simulink model "doc_commmsksync"  (R2014a)
settings: Solver=FixedStepDiscrete  SolverMode=SingleTasking  StartTime=0.0  StopTime=2.0  RelTol=1e-3
model workspace (MATLAB code in the model file):
  | tsym = 1/280000;
  | sampPerSymb = 14;
  | trDepth = 16;
libraries: dspsigops x5, dspstat3 x2, commutil2 x2, simulink_extras x2, commdigbbndcpm2 x2, commsink2 x1, commblksprivate x1, commfilt2 x1, dspmathops x1, dspmtrx3 x1, commchan3 x1, commrflib2 x1
CloseFcn:
  | if exist('commmsksync_sigsOut','var'), clear commmsksync_sigsOut; end;
Description:
  | MSK Signal:  Timing, Carrier Frequency and Carrier Phase Recovery
  | 
  | This model shows the modeling of channel impairments such as timing phase offset, carrier frequency, and phase offsets for a minimum shift keying (MSK) signal.
settings Model: ExtModeAutoUpdateStatusClock=off  Creator=The MathWorks Inc.
settings DataIOCC: LimitDataPoints=off  SignalLoggingSaveFormat=ModelDataLogs  SaveOutput=off  SaveTime=off  SignalLoggingName=commmsksync_sigsOut
settings OptimizationCC: BooleanDataType=off  ExpressionDepthLimit=2147483647  InitFltsAndDblsToZero=on  EfficientMapNaN2IntZero=off
settings DebuggingCC: SaveWithParameterizedLinksMsg=none  UnderspecifiedInitializationDetection=Classic  CheckExecutionContextPreStartOutputMsg=on  CheckExecutionContextRuntimeOutputMsg=on  SignalResolutionControl=TryResolveAllWithWarning  SolverPrmCheckMsg=none  InheritedTsInSrcMsg=none  MultiTaskDSMMsg=warning  MultiTaskCondExecSysMsg=none  SigSpecEnsureSampleTimeMsg=none  FcnCallInpInsideContextMsg=UseLocalSettings  StateNameClashWarn=warning  StrictBusMsg=None
settings HardwareCC: ProdHWDeviceType=Specified
settings ModelReferenceCC: UpdateModelReferenceTargets=IfOutOfDate
settings RTWCC: IncludeERTFirstTime=on
settings GRTTargetCC: TargetFcnLib=ansi_tfl_tmw.mat  CombineOutputUpdateFcns=off  GRTInterface=on

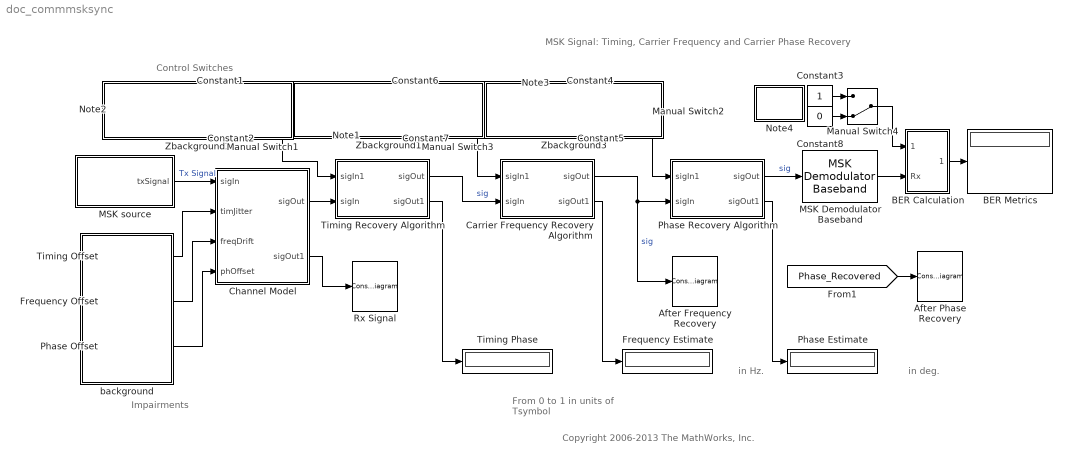
== system doc_commmsksync ==
  note: MSK Signal:
      | Timing, Carrier Frequency and Carrier Phase Recovery
  note: in Hz.
  note: From 0 to 1
      | in units of Tsymbol
  note: in deg.
  note: Control Switches
  note: Impairments
  note: Copyright 2006-2013 The MathWorks, Inc.
  After Frequency Recovery : ConstellationDiagram  Tag=ScatterPlot
  After Phase Recovery : ConstellationDiagram  Tag=ScatterPlot
  BER Calculation : Subsystem
      mask Display: disp('BER')
  BER Metrics : Display
  Carrier Frequency Recovery Algorithm : Subsystem  mask(Carrier Frequency Recovery algorithm){}
      mask Display: disp('Carrier Freq.\nRecovery')
  Channel Model : Subsystem  mask(RF Impairments){}
      mask Display: plot(-10,-10,110, 110,[05 15 10 10 05 10 18 14 13 7.5 13 41 44 47 50 53 57 59 100-[13 7.5 13 14 18 10 5 10 10 15 5]],[70 70 70 85 92 85 79 82 90 88.5 90 90 87 93 87 93 87 90 90 88.5 90 82 79 85 92 85 70 70 70]-30);
  Constant{1,3..4,6} (4 alike) : Constant  SampleTime=tsym*1000
  Constant{2,5,7..8} (4 alike) : Constant  Value=0  SampleTime=tsym*1000
  Frequency Estimate : Display
  Frequency Offset : Constant  Value=50
  MSK Demodulator Baseband : commdigbbndcpm2/MSK Demodulator Baseband  outputType=Bit  phaseOffset=0  samplesPerSymbol=1  RateOptions=Enforce single-rate processing  traceBack=trDepth  outDType=double
  MSK source : Subsystem  mask(GMSK source){}
      mask Display: disp('MSK\nSource')
  Manual Switch1 : ManualSwitch
  Manual Switch2 : ManualSwitch
  Manual Switch3 : ManualSwitch
  Manual Switch4 : ManualSwitch  CurrentSetting=0
  Note1 : Subsystem
      mask Display: disp('Carrier Frequency\nRecovery')
  Note2 : Subsystem
      mask Display: disp('Timing Phase\nRecovery')
  Note3 : Subsystem
      mask Display: disp('Phase\nRecovery')
  Note4 : Subsystem
      mask Display: disp('Reset\nBER')
  Phase Estimate : Display
  Phase Offset : Constant  Value=30
  Phase Recovery Algorithm : Subsystem  mask(Carrier Frequency Recovery algorithm){}
      mask Display: disp('Phase\nRecovery')
  Rx Signal : ConstellationDiagram  Tag=ScatterPlot
  Timing Offset : Constant  Value=0.2
  Timing Phase : Display
  Timing Recovery Algorithm : Subsystem  mask(Timing recovery algorithm.){}
      mask Display: disp('Timing\nRecovery');
  Zbackground1 : Subsystem
      mask Display: disp('')
  Zbackground2 : Subsystem
      mask Display: disp('')
  Zbackground3 : Subsystem
      mask Display: disp('')
  background : Subsystem
      mask Display: disp('')
  wires:
  Carrier Frequency Recovery Algorithm/1(sigOut) -> Phase Recovery Algorithm/2(sigIn), After Frequency Recovery/1  "sig"
  MSK source/1(txSignal) -> Channel Model/1(sigIn)  "Tx Signal"
  Channel Model/1(sigOut) -> Timing Recovery Algorithm/2(sigIn)
  Manual Switch1/1 -> Timing Recovery Algorithm/1(sigIn1)
  Timing Recovery Algorithm/1(sigOut) -> Carrier Frequency Recovery Algorithm/2(sigIn)  "sig"
  Manual Switch3/1 -> Carrier Frequency Recovery Algorithm/1(sigIn1)
  Timing Offset/1 -> Channel Model/2(timJitter)
  Frequency Offset/1 -> Channel Model/3(freqDrift)
  Timing Recovery Algorithm/2(sigOut1) -> Timing Phase/1
  Carrier Frequency Recovery Algorithm/2(sigOut1) -> Frequency Estimate/1
  Phase Recovery Algorithm/2(sigOut1) -> Phase Estimate/1
  Phase Offset/1 -> Channel Model/4(phOffset)
  Phase Recovery Algorithm/1(sigOut) -> MSK Demodulator Baseband/1  "sig"
  MSK Demodulator Baseband/1 -> BER Calculation/2(Rx)
  BER Calculation/1(Out1) -> BER Metrics/1
  Channel Model/2(sigOut1) -> Rx Signal/1
  Manual Switch4/1 -> BER Calculation/1(Rst)
  [Phase_Recovered] -> After Phase Recovery/1
  Manual Switch2/1 -> Phase Recovery Algorithm/1(sigIn1)
  Constant4/1 -> Manual Switch2/1
  Constant5/1 -> Manual Switch2/2
  Constant6/1 -> Manual Switch3/1
  Constant7/1 -> Manual Switch3/2
  Constant1/1 -> Manual Switch1/1
  Constant2/1 -> Manual Switch1/2
  Constant3/1 -> Manual Switch4/1
  Constant8/1 -> Manual Switch4/2

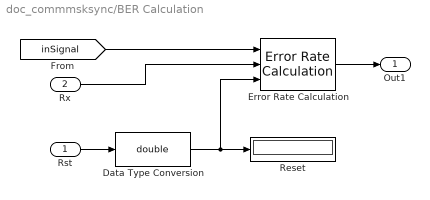
== system doc_commmsksync/BER Calculation ==
  Rst : Inport
  Rx : Inport  Port=2
  Data Type Conversion : DataTypeConversion  OutDataTypeStr=double
  Error Rate Calculation : commsink2/Error Rate Calculation  N=trDepth+2 % Traceback Depth + Delay due to Timing Recovery  st_delay=0  cp_mode=Entire frame  subframe=[]  PMode=Port  WsName=ErrorVec  RsMode2=on  stop=off  numErr=100  maxBits=1e6
  Reset : Display
  Out1 : Outport
  wires:
  Error Rate Calculation/1 -> Out1/1
  Rst/1 -> Data Type Conversion/1
  Data Type Conversion/1 -> Reset/1, Error Rate Calculation/3
  Rx/1 -> Error Rate Calculation/2
  [inSignal] -> Error Rate Calculation/1

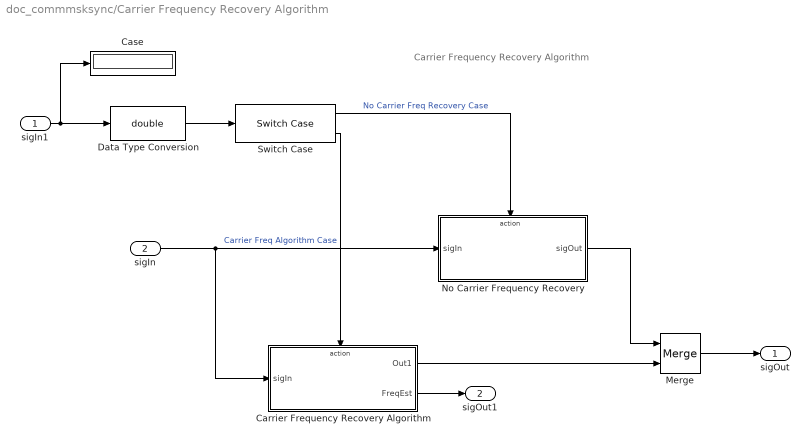
== system doc_commmsksync/Carrier Frequency Recovery Algorithm ==
  note: Carrier Frequency Recovery Algorithm
  sigIn1 : Inport
  sigIn : Inport  Port=2
  Carrier Frequency Recovery Algorithm : Subsystem  TreatAsAtomicUnit=on
  Case : Display
  Data Type Conversion : DataTypeConversion  OutDataTypeStr=double
  Merge : Merge
  No Carrier Frequency Recovery : Subsystem  TreatAsAtomicUnit=on
  Switch Case : SwitchCase  CaseConditions={0,1}  ShowDefaultCase=off
  sigOut : Outport
  sigOut1 : Outport  Port=2
  wires:
  sigIn/1 -> No Carrier Frequency Recovery/1(sigIn), Carrier Frequency Recovery Algorithm/1(sigIn)
  Merge/1 -> sigOut/1
  Switch Case/2 -> Carrier Frequency Recovery Algorithm/Action  "Carrier Freq Algorithm Case"
  Switch Case/1 -> No Carrier Frequency Recovery/Action  "No Carrier Freq Recovery Case"
  No Carrier Frequency Recovery/1(sigOut) -> Merge/1
  Carrier Frequency Recovery Algorithm/1(Out1) -> Merge/2
  Carrier Frequency Recovery Algorithm/2(FreqEst) -> sigOut1/1
  sigIn1/1 -> Data Type Conversion/1, Case/1
  Data Type Conversion/1 -> Switch Case/1

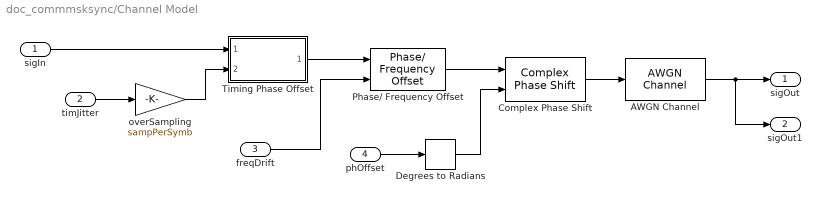
== system doc_commmsksync/Channel Model ==
  sigIn : Inport
  timJitter : Inport  Port=2
  freqDrift : Inport  Port=3
  phOffset : Inport  Port=4
  AWGN Channel : commchan3/AWGN Channel  InputProcessing=Columns as channels (frame based)  seed=67  noiseMode="Signal to noise ratio  (Eb/No)"  EbNodB=60  EsNodB=10  SNRdB=10  bitsPerSym=1  Ps=1  Tsym=tsym  variance=1
  Complex Phase Shift : commutil2/Complex Phase Shift
  Degrees to Radians : simulink_extras/Transformations/Degrees to Radians
  Phase/ Frequency Offset : commrflib2/Phase// Frequency Offset  phaseOffset=0  freqPort=on  freqOffset=0
  Timing Phase Offset : Subsystem
      mask Display: disp('Timing Phase\nOffset')
  overSampling : Gain  Gain=sampPerSymb  SaturateOnIntegerOverflow=on  OutDataTypeStr=Inherit: Same as input  ParamDataTypeStr=Inherit: Same as input
  sigOut : Outport
  sigOut1 : Outport  Port=2
  wires:
  AWGN Channel/1 -> sigOut/1, sigOut1/1
  sigIn/1 -> Timing Phase Offset/1(InSignal)
  timJitter/1 -> overSampling/1
  Timing Phase Offset/1(OutSignal) -> Phase/ Frequency Offset/1
  overSampling/1 -> Timing Phase Offset/2(phOffset)
  freqDrift/1 -> Phase/ Frequency Offset/2
  Phase/ Frequency Offset/1 -> Complex Phase Shift/1
  Complex Phase Shift/1 -> AWGN Channel/1
  Degrees to Radians/1 -> Complex Phase Shift/2
  phOffset/1 -> Degrees to Radians/1

== system doc_commmsksync/MSK source ==
  note: in bps.
  Bernoulli Binary Generator : commrandsrc2/Bernoulli Binary Generator  P=0.5  seed=61  Ts=tsym  frameBased=on  sampPerFrame=1000  orient=off  outDataType=double
  Compute Bit Rate : Subsystem  mask(Compute bit rate of signal){overSamp=sampPerSymb}
      mask prompts: overSamp "Oversampling factor:"
      mask help: Bit rate calculation based on probed sample time and a specified number of bits per sample.
      mask Display: disp('Compute\nBit Rate')
  MSK Modulator Baseband : commdigbbndcpm2/MSK Modulator Baseband  inputType=Bit  phaseOffset=0  samplesPerSymbol=sampPerSymb  RateOptions=Enforce single-rate processing  outDataType=double
  bit rate : Display
  txSignal : Outport
  tag scope: inSignal=global
  wires:
  Bernoulli Binary Generator/1 -> [inSignal], MSK Modulator Baseband/1
  MSK Modulator Baseband/1 -> Compute Bit Rate/1(sig), txSignal/1
  Compute Bit Rate/1(rate) -> bit rate/1

== system doc_commmsksync/Note1 ==

== system doc_commmsksync/Note2 ==

== system doc_commmsksync/Note3 ==

== system doc_commmsksync/Note4 ==

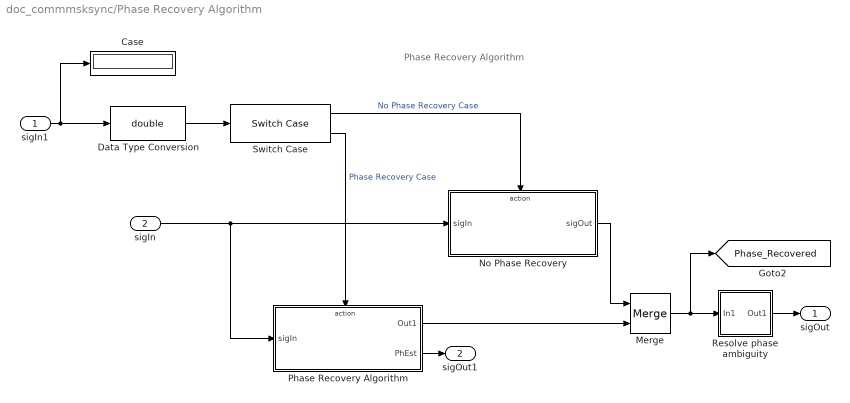
== system doc_commmsksync/Phase Recovery Algorithm ==
  note: Phase Recovery Algorithm
  sigIn1 : Inport
  sigIn : Inport  Port=2
  Case : Display
  Data Type Conversion : DataTypeConversion  OutDataTypeStr=double
  Merge : Merge
  No Phase Recovery : Subsystem  TreatAsAtomicUnit=on
  Phase Recovery Algorithm : Subsystem  TreatAsAtomicUnit=on
  Resolve phase ambiguity : Subsystem
  Switch Case : SwitchCase  CaseConditions={0,1}  ShowDefaultCase=off
  sigOut : Outport
  sigOut1 : Outport  Port=2
  tag scope: Phase_Recovered=global
  wires:
  Data Type Conversion/1 -> Switch Case/1
  sigIn1/1 -> Case/1, Data Type Conversion/1
  Phase Recovery Algorithm/2(PhEst) -> sigOut1/1
  Phase Recovery Algorithm/1(Out1) -> Merge/2
  No Phase Recovery/1(sigOut) -> Merge/1
  Switch Case/1 -> No Phase Recovery/Action  "No Phase Recovery Case"
  Switch Case/2 -> Phase Recovery Algorithm/Action  "Phase Recovery Case"
  Merge/1 -> Resolve phase ambiguity/1(In1), [Phase_Recovered]
  sigIn/1 -> Phase Recovery Algorithm/1(sigIn), No Phase Recovery/1(sigIn)
  Resolve phase ambiguity/1(Out1) -> sigOut/1

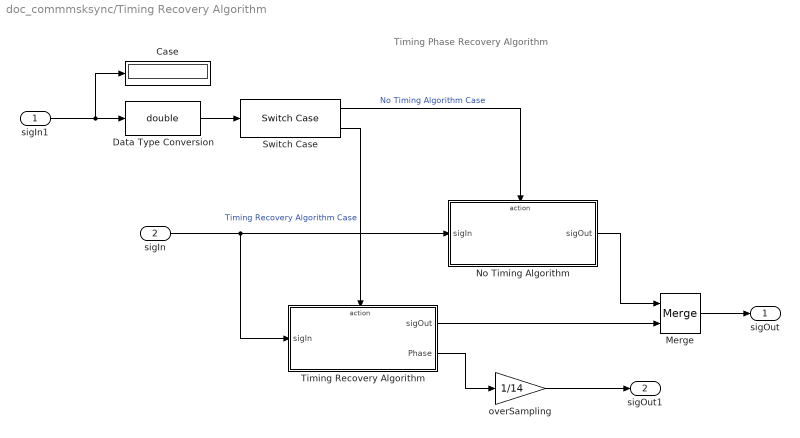
== system doc_commmsksync/Timing Recovery Algorithm ==
  note: Timing Phase Recovery Algorithm
  sigIn1 : Inport
  sigIn : Inport  Port=2
  Case : Display
  Data Type Conversion : DataTypeConversion  OutDataTypeStr=double
  Merge : Merge
  No Timing Algorithm : Subsystem  TreatAsAtomicUnit=on
  Switch Case : SwitchCase  CaseConditions={0,1}  ShowDefaultCase=off
  Timing Recovery Algorithm : Subsystem  TreatAsAtomicUnit=on
  overSampling : Gain  Gain=1/14  SaturateOnIntegerOverflow=on  OutDataTypeStr=Inherit: Same as input  ParamDataTypeStr=Inherit: Same as input
  sigOut : Outport
  sigOut1 : Outport  Port=2
  wires:
  sigIn/1 -> Timing Recovery Algorithm/1(sigIn), No Timing Algorithm/1(sigIn)
  Merge/1 -> sigOut/1
  Switch Case/2 -> Timing Recovery Algorithm/Action  "Timing Recovery Algorithm Case"
  Switch Case/1 -> No Timing Algorithm/Action  "No Timing Algorithm Case"
  No Timing Algorithm/1(sigOut) -> Merge/1
  Timing Recovery Algorithm/1(sigOut) -> Merge/2
  Timing Recovery Algorithm/2(Phase) -> overSampling/1
  sigIn1/1 -> Data Type Conversion/1, Case/1
  overSampling/1 -> sigOut1/1
  Data Type Conversion/1 -> Switch Case/1

== system doc_commmsksync/Zbackground1 ==
  note: This subsystem is empty

== system doc_commmsksync/Zbackground2 ==
  note: This subsystem is empty

== system doc_commmsksync/Zbackground3 ==
  note: This subsystem is empty

== system doc_commmsksync/background ==
  note: This subsystem is empty

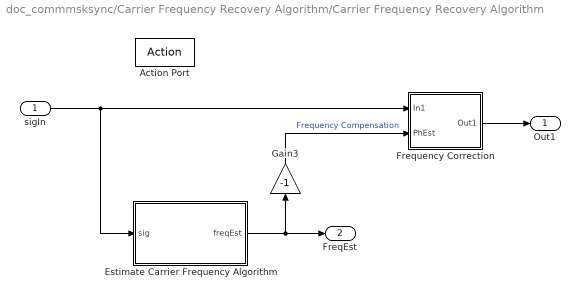
== system doc_commmsksync/Carrier Frequency Recovery Algorithm/Carrier Frequency Recovery Algorithm ==
  sigIn : Inport
  Action Port : ActionPort  InitializeStates=reset  PropagateVarSize=During execution  ActionType=case
  Estimate Carrier Frequency Algorithm : Subsystem
  Frequency Correction : Subsystem
      mask Display: disp('Frequency\nCorrection');
  Gain3 : Gain  Gain=-1  SaturateOnIntegerOverflow=on  OutDataTypeStr=Inherit: Same as input  ParamDataTypeStr=Inherit: Same as input
  Out1 : Outport
  FreqEst : Outport  Port=2  OutputWhenDisabled=reset  InitialOutput=0
  wires:
  sigIn/1 -> Estimate Carrier Frequency Algorithm/1(sig), Frequency Correction/1(In1)
  Frequency Correction/1(Out1) -> Out1/1
  Gain3/1 -> Frequency Correction/2(PhEst)  "Frequency Compensation"
  Estimate Carrier Frequency Algorithm/1(freqEst) -> FreqEst/1, Gain3/1

== system doc_commmsksync/Carrier Frequency Recovery Algorithm/No Carrier Frequency Recovery ==
  sigIn : Inport
  Action Port : ActionPort  PropagateVarSize=During execution  ActionType=case
  sigOut : Outport
  wires:
  sigIn/1 -> sigOut/1

== system doc_commmsksync/Channel Model/Timing Phase Offset ==
  InSignal : Inport
  phOffset : Inport  Port=2
  Variable Fractional Delay : dspsigops/Variable Fractional Delay  mode=OBSOLETE  modeActive=Linear  dmax=100  InputProcessing=Columns as channels (frame based)  L=4  FarrowL=4  R=10  alpha=1  ic=0  fallbackFIR=Clip to the minimum value necessary for centered kernel  fallbackFarrow=Clip to the minimum value necessary for centered kernel  noDFT=off  roundingMode=Zero  overflowMode=off
  OutSignal : Outport
  wires:
  Variable Fractional Delay/1 -> OutSignal/1
  InSignal/1 -> Variable Fractional Delay/1
  phOffset/1 -> Variable Fractional Delay/2

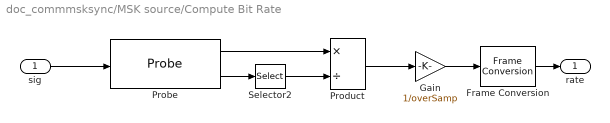
== system doc_commmsksync/MSK source/Compute Bit Rate ==
  sig : Inport
  Frame Conversion : FrameConversion
  Gain : Gain  Gain=1/overSamp  SaturateOnIntegerOverflow=on  OutDataTypeStr=Inherit: Same as input  ParamDataTypeStr=Inherit: Same as input
  Probe : Probe  ProbeComplexSignal=off
  Product : Product  Inputs=*/  SaturateOnIntegerOverflow=on  InputSameDT=on  OutDataTypeStr=Inherit: Same as first input
  Selector2 : Selector  InputPortWidth=2  Indices=[1 ]
  rate : Outport
  wires:
  Product/1 -> Gain/1
  sig/1 -> Probe/1
  Selector2/1 -> Product/2
  Probe/2 -> Selector2/1
  Probe/1 -> Product/1
  Gain/1 -> Frame Conversion/1
  Frame Conversion/1 -> rate/1

== system doc_commmsksync/Phase Recovery Algorithm/No Phase Recovery ==
  sigIn : Inport
  Action Port : ActionPort  PropagateVarSize=During execution  ActionType=case
  sigOut : Outport
  wires:
  sigIn/1 -> sigOut/1

== system doc_commmsksync/Phase Recovery Algorithm/Phase Recovery Algorithm ==
  sigIn : Inport
  Action Port : ActionPort  InitializeStates=reset  PropagateVarSize=During execution  ActionType=case
  CPM Phase Recovery : commphrec2/CPM Phase Recovery  P=2  intPeriod=1000
  Out1 : Outport
  PhEst : Outport  Port=2  OutputWhenDisabled=reset  InitialOutput=0
  wires:
  sigIn/1 -> CPM Phase Recovery/1
  CPM Phase Recovery/1 -> Out1/1
  CPM Phase Recovery/2 -> PhEst/1

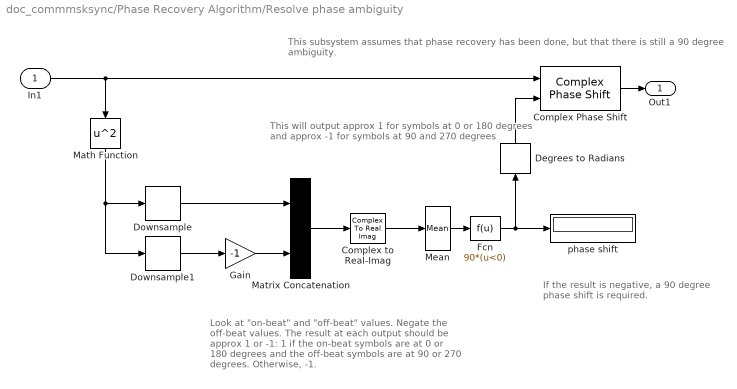
== system doc_commmsksync/Phase Recovery Algorithm/Resolve phase ambiguity ==
  note: If the result is negative,
      | a 90 degree phase shift is required.
  note: Look at "on-beat" and "off-beat" values.
      | Negate the off-beat values.
      | The result at each output should be approx 1 or -1:
      | 1 if the on-beat symbols are at 0 or 180 degrees
      | and the off-beat symbols are at 90 or 270 degrees.
      | Otherwise, -1.
  note: This will output approx 1 for symbols at 0 or 180 degrees
      | and approx -1 for symbols at 90 and 270 degrees
  note: This subsystem assumes that phase recovery has been done, but that there is still a 90 degree ambiguity.
  In1 : Inport
  Complex Phase Shift : commutil2/Complex Phase Shift
  Complex to Real-Imag : ComplexToRealImag  Output=Real
  Degrees to Radians : simulink_extras/Transformations/Degrees to Radians
  Downsample : dspsigops/Downsample  N=2  phase=0  InputProcessing=Columns as channels (frame based)  RateOptions=Enforce single-rate processing  smode=Allow multirate  fmode=Maintain input frame rate  ic=0
  Downsample1 : dspsigops/Downsample  N=2  phase=1  InputProcessing=Columns as channels (frame based)  RateOptions=Enforce single-rate processing  smode=Allow multirate  fmode=Maintain input frame rate  ic=0
  Fcn : Fcn  Expr=90*(u<0)
  Gain : Gain  Gain=-1
  Math Function : Math  Operator=square  SaturateOnIntegerOverflow=on
  Matrix Concatenation : Concatenate  Mode=Multidimensional array
  Mean : dspstat3/Mean  run=off  reset_popup=None  InputProcessing=Columns as channels (frame based)  directionMode=Each column  dimension=1  treatSBRowAsCol=on  roiEnable=off  roiType=Rectangles  roiPortion=Entire ROI  roiOutput=Individual statistics for each ROI  roiFlag=off  outputDataTypeStr=Inherit: Same as accumulator  outputLastDataTypeStr=Inherit: Same as accumulator  outputMin=[]  outputMax=[]  roundingMode=Floor  overflowMode=off
  phase shift : Display
  Out1 : Outport
  wires:
  Fcn/1 -> phase shift/1, Degrees to Radians/1
  Complex to Real-Imag/1 -> Mean/1
  Mean/1 -> Fcn/1
  Matrix Concatenation/1 -> Complex to Real-Imag/1
  Gain/1 -> Matrix Concatenation/2
  Downsample1/1 -> Gain/1
  Downsample/1 -> Matrix Concatenation/1
  Math Function/1 -> Downsample1/1, Downsample/1
  Complex Phase Shift/1 -> Out1/1
  In1/1 -> Math Function/1, Complex Phase Shift/1
  Degrees to Radians/1 -> Complex Phase Shift/2

== system doc_commmsksync/Timing Recovery Algorithm/No Timing Algorithm ==
  sigIn : Inport
  Action Port : ActionPort  PropagateVarSize=During execution  ActionType=case
  Downsample : dspsigops/Downsample  N=14  phase=0  InputProcessing=Columns as channels (frame based)  RateOptions=Enforce single-rate processing  smode=Allow multirate  fmode=Maintain input frame rate  ic=0
  sigOut : Outport
  wires:
  sigIn/1 -> Downsample/1
  Downsample/1 -> sigOut/1

== system doc_commmsksync/Timing Recovery Algorithm/Timing Recovery Algorithm ==
  note: The Sym output is the result of applying the
      | estimated phase correction to the input signal.
  note: The Ph output gives the phase estimate
      | for each symbol in the input signal.
  sigIn : Inport
  Action Port : ActionPort  InitializeStates=reset  PropagateVarSize=During execution  ActionType=case
  MSK-Type Signal Timing Recovery : commtimrec2/MSK-Type Signal Timing Recovery  modType=MSK  sampPerSymbol=sampPerSymb  propGain=0.2  resetMode=None
  Multiport Selector : dspindex/Multiport Selector  rowsOrCols=Rows  idxCellArray={1}  idxErrMode=Clip Index
  sigOut : Outport
  Phase : Outport  Port=2  OutputWhenDisabled=reset  InitialOutput=0
  wires:
  sigIn/1 -> MSK-Type Signal Timing Recovery/1
  MSK-Type Signal Timing Recovery/1 -> sigOut/1
  MSK-Type Signal Timing Recovery/2 -> Multiport Selector/1
  Multiport Selector/1 -> Phase/1

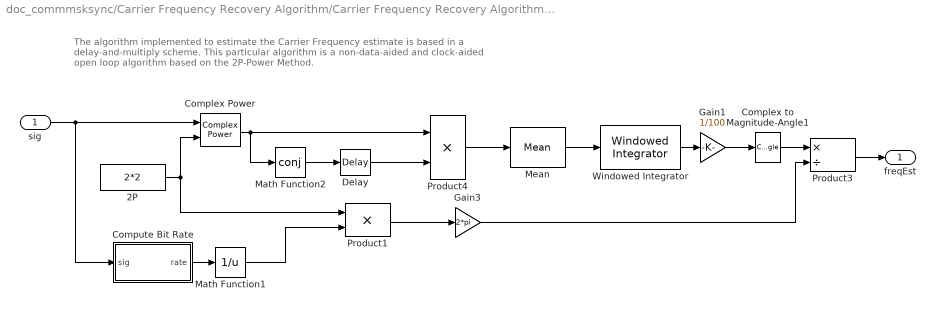
== system doc_commmsksync/Carrier Frequency Recovery Algorithm/Carrier Frequency Recovery Algorithm/Estimate Carrier Frequency Algorithm ==
  note: The algorithm implemented to estimate the Carrier Frequency estimate is based in a
      | delay-and-multiply scheme. This particular algorithm is a non-data-aided
      | and clock-aided open loop algorithm based on the 2P-Power Method.
  sig : Inport
  2P : Constant  Value=2*2
  Complex Power : commblksprivate/Complex Power
  Complex to Magnitude-Angle1 : ComplexToMagnitudeAngle  Output=Angle
  Compute Bit Rate : Subsystem  mask(Compute bit rate of signal){overSamp=1}
      mask prompts: overSamp "Oversampling factor:"
      mask help: Bit rate calculation based on probed sample time and a specified number of bits per sample.
      mask Display: disp('Compute\nBit Rate')
  Delay : dspsigops/Delay  InputProcessing=Columns as channels (frame based)  dly_unit=Samples  delay=1  ic_detail=off  dif_ic_for_ch=off  dif_ic_for_dly=off  ic=0  reset_popup=None
  Gain1 : Gain  Gain=1/100  SaturateOnIntegerOverflow=on  OutDataTypeStr=Inherit: Same as input  ParamDataTypeStr=Inherit: Same as input
  Gain3 : Gain  Gain=2*pi  SaturateOnIntegerOverflow=on  OutDataTypeStr=Inherit: Same as input  ParamDataTypeStr=Inherit: Same as input
  Math Function1 : Math  Operator=reciprocal  SaturateOnIntegerOverflow=on
  Math Function2 : Math  Operator=conj  SaturateOnIntegerOverflow=on
  Mean : dspstat3/Mean  run=off  reset_popup=None  InputProcessing=Columns as channels (frame based)  directionMode=Each column  dimension=1  treatSBRowAsCol=on  roiEnable=off  roiType=Rectangles  roiPortion=Entire ROI  roiOutput=Individual statistics for each ROI  roiFlag=off  outputDataTypeStr=Inherit: Same as accumulator  outputLastDataTypeStr=Inherit: Same as accumulator  outputMin=[]  outputMax=[]  roundingMode=Floor  overflowMode=off
  Product1 : Product  Inputs=**  SaturateOnIntegerOverflow=on  OutDataTypeStr=Inherit: Same as first input
  Product3 : Product  Inputs=*/  SaturateOnIntegerOverflow=on  OutDataTypeStr=Inherit: Same as first input
  Product4 : Product  SaturateOnIntegerOverflow=on  OutDataTypeStr=Inherit: Same as first input
  Windowed Integrator : commfilt2/Windowed Integrator  integperiod=100  roundingMode=Floor  overflowMode=off  InputProcessing=Columns as channels (frame based)
  freqEst : Outport
  wires:
  Product1/1 -> Gain3/1
  2P/1 -> Product1/1, Complex Power/2
  Complex Power/1 -> Product4/1, Math Function2/1
  Math Function2/1 -> Delay/1
  Delay/1 -> Product4/2
  Product4/1 -> Mean/1
  Complex to Magnitude-Angle1/1 -> Product3/1
  Gain3/1 -> Product3/2
  sig/1 -> Compute Bit Rate/1(sig), Complex Power/1
  Product3/1 -> freqEst/1
  Mean/1 -> Windowed Integrator/1
  Compute Bit Rate/1(rate) -> Math Function1/1
  Math Function1/1 -> Product1/2
  Gain1/1 -> Complex to Magnitude-Angle1/1
  Windowed Integrator/1 -> Gain1/1

== system doc_commmsksync/Carrier Frequency Recovery Algorithm/Carrier Frequency Recovery Algorithm/Frequency Correction ==
  In1 : Inport
  PhEst : Inport  Port=2
  Calculate Frequency Offset : Subsystem
      mask Display: disp('Calculate\nFrequency\nOffset');
  Product : Product  SaturateOnIntegerOverflow=on  InputSameDT=on  OutDataTypeStr=Inherit: Same as first input
  Out1 : Outport
  wires:
  Calculate Frequency Offset/1(Out1) -> Product/2
  In1/1 -> Calculate Frequency Offset/1(In1), Product/1
  Product/1 -> Out1/1
  PhEst/1 -> Calculate Frequency Offset/2(Freq)

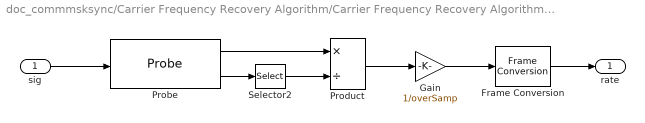
== system doc_commmsksync/Carrier Frequency Recovery Algorithm/Carrier Frequency Recovery Algorithm/Estimate Carrier Frequency Algorithm/Compute Bit Rate ==
  sig : Inport
  Frame Conversion : FrameConversion
  Gain : Gain  Gain=1/overSamp  SaturateOnIntegerOverflow=on  OutDataTypeStr=Inherit: Same as input  ParamDataTypeStr=Inherit: Same as input
  Probe : Probe  ProbeComplexSignal=off
  Product : Product  Inputs=*/  SaturateOnIntegerOverflow=on  InputSameDT=on  OutDataTypeStr=Inherit: Same as first input
  Selector2 : Selector  InputPortWidth=2  Indices=[1 ]
  rate : Outport
  wires:
  Product/1 -> Gain/1
  sig/1 -> Probe/1
  Selector2/1 -> Product/2
  Probe/2 -> Selector2/1
  Probe/1 -> Product/1
  Gain/1 -> Frame Conversion/1
  Frame Conversion/1 -> rate/1

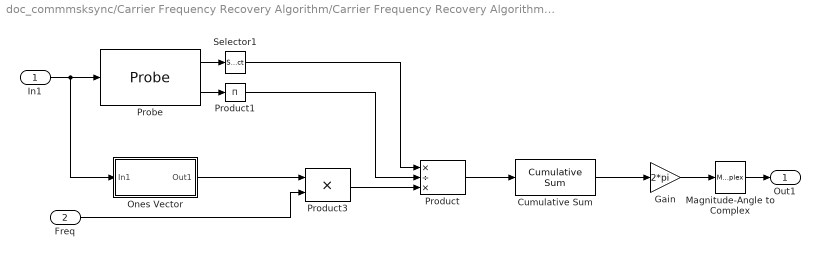
== system doc_commmsksync/Carrier Frequency Recovery Algorithm/Carrier Frequency Recovery Algorithm/Frequency Correction/Calculate Frequency Offset ==
  In1 : Inport
  Freq : Inport  Port=2
  Cumulative Sum : dspmathops/Cumulative Sum  dim=Channels (running sum)  InputProcessing=Columns as channels (frame based)  reset_popup=None  outputDataTypeStr=Inherit: Same as accumulator  outputLastDataTypeStr=Inherit: Same as accumulator  outputMin=[]  outputMax=[]  roundingMode=Floor  overflowMode=off
  Gain : Gain  Gain=2*pi  SaturateOnIntegerOverflow=on  OutDataTypeStr=Inherit: Same as input  ParamDataTypeStr=Inherit: Same as input
  Magnitude-Angle to Complex : MagnitudeAngleToComplex  Input=Angle  ConstantPart=1
  Ones Vector : Subsystem  mask(Ones Vector){}
      mask help: Create a vector of equals whose length is equal to input portwidth.
      mask Display: disp('Ones(1:length)')
  Probe : Probe  ProbeWidth=off  ProbeComplexSignal=off  ProbeSignalDimensions=on
  Product : Product  Inputs=*/*  SaturateOnIntegerOverflow=on  InputSameDT=on  OutDataTypeStr=Inherit: Same as first input
  Product1 : Product  Inputs=1  SaturateOnIntegerOverflow=on  InputSameDT=on  OutDataTypeStr=Inherit: Same as first input
  Product3 : Product  Inputs=**  SaturateOnIntegerOverflow=on  OutDataTypeStr=Inherit: Same as first input
  Selector1 : Selector  InputPortWidth=2  Indices=[1 ]
  Out1 : Outport
  wires:
  Selector1/1 -> Product/1
  Product1/1 -> Product/2
  Probe/1 -> Selector1/1
  Product/1 -> Cumulative Sum/1
  Probe/2 -> Product1/1
  In1/1 -> Probe/1, Ones Vector/1(In1)
  Magnitude-Angle to Complex/1 -> Out1/1
  Gain/1 -> Magnitude-Angle to Complex/1
  Product3/1 -> Product/3
  Freq/1 -> Product3/2
  Cumulative Sum/1 -> Gain/1
  Ones Vector/1(Out1) -> Product3/1

== system doc_commmsksync/Carrier Frequency Recovery Algorithm/Carrier Frequency Recovery Algorithm/Frequency Correction/Calculate Frequency Offset/Ones Vector ==
  In1 : Inport
  Bias : dspmtrx3/Array-Vector Add  Dimension=2  V_Source=Dialog parameter  V_VectFromMask=1  firstCoeffSignedness=Auto  firstCoeffDataTypeStr=Inherit: Same word length as input  firstCoeffLastDataTypeStr=Inherit: Same word length as input  firstCoeffMin=[]  firstCoeffMax=[]  outputSignedness=Auto  outputMin=[]  outputMax=[]  accumSignedness=Auto  prodOutputSignedness=Auto  roundingMode=Floor  overflowMode=off
  Complex to Real-Imag : ComplexToRealImag  Output=Real
  Gain1 : Gain  Gain=0
  Out1 : Outport
  wires:
  Complex to Real-Imag/1 -> Gain1/1
  Gain1/1 -> Bias/1
  In1/1 -> Complex to Real-Imag/1
  Bias/1 -> Out1/1
